simulink library "halin"  (R2021b)
settings: Solver=VariableStepAuto  StartTime=0.0  StopTime=10.0  RelTol=1e-3
undefined symbols (not defined in the file): TRUE
libraries: FVT_lib x177, hcu_lib x55
(part 15 of 17)

== system halin/HAL_IN/CAN3/MCU_B_R1/RrMCUDCBusCurr ==
  Rr_MCUDCBusCurr : Inport
  UnitConverter : DataTypeConversion  OutDataTypeStr=uint16
  convert_in : FVT_lib/hal/convert_in  gain=0.1  offset=-1500
  VHAL_RrMCUDCBusCurr_A : Outport
  wires:
  convert_in/1 -> VHAL_RrMCUDCBusCurr_A/1
  UnitConverter/1 -> convert_in/1
  Rr_MCUDCBusCurr/1 -> UnitConverter/1

== system halin/HAL_IN/CAN3/MCU_B_R1/RrMCUDCBusVolt ==
  Rr_MCUDCBusVolt : Inport
  UnitConverter : DataTypeConversion  OutDataTypeStr=uint16
  convert_in : FVT_lib/hal/convert_in  gain=0.1  offset=0
  VHAL_RrMCUDCBusVolt_V : Outport
  wires:
  convert_in/1 -> VHAL_RrMCUDCBusVolt_V/1
  UnitConverter/1 -> convert_in/1
  Rr_MCUDCBusVolt/1 -> UnitConverter/1

== system halin/HAL_IN/CAN3/MCU_B_R1/RrMCUDischrgSta ==
  Rr_MCUDischrgSta : Inport
  UnitConverter : DataTypeConversion  OutDataTypeStr=uint8
  VHAL_RrMCUDischrgSta_flg : Outport
  wires:
  UnitConverter/1 -> VHAL_RrMCUDischrgSta_flg/1
  Rr_MCUDischrgSta/1 -> UnitConverter/1

== system halin/HAL_IN/CAN3/MCU_B_R1/RrMCUEnaSta ==
  Rr_MCUEnaSta : Inport
  UnitConverter : DataTypeConversion  OutDataTypeStr=uint8
  VHAL_RrMCUEnaSta_flg : Outport
  wires:
  UnitConverter/1 -> VHAL_RrMCUEnaSta_flg/1
  Rr_MCUEnaSta/1 -> UnitConverter/1

== system halin/HAL_IN/CAN3/MCU_B_R1/RrMCUErr ==
  Rr_MCUErr : Inport
  UnitConverter : DataTypeConversion  OutDataTypeStr=uint8
  VHAL_RrMCUErr_enum : Outport
  wires:
  UnitConverter/1 -> VHAL_RrMCUErr_enum/1
  Rr_MCUErr/1 -> UnitConverter/1

== system halin/HAL_IN/CAN3/MCU_B_R1/RrMCUIGNsta ==
  Rr_MCUIGN_sta : Inport
  UnitConverter : DataTypeConversion  OutDataTypeStr=uint8
  VHAL_RrMCUIGNsta_flg : Outport
  wires:
  UnitConverter/1 -> VHAL_RrMCUIGNsta_flg/1
  Rr_MCUIGN_sta/1 -> UnitConverter/1

== system halin/HAL_IN/CAN3/MCU_B_R1/RrMCUReady ==
  Rr_MCUReady : Inport
  UnitConverter : DataTypeConversion  OutDataTypeStr=uint8
  VHAL_RrMCUReady_flg : Outport
  wires:
  UnitConverter/1 -> VHAL_RrMCUReady_flg/1
  Rr_MCUReady/1 -> UnitConverter/1

== system halin/HAL_IN/CAN3/MCU_B_R1/RrMCUReady4Pre ==
  Rr_MCUReady4Pre : Inport
  UnitConverter : DataTypeConversion  OutDataTypeStr=uint8
  VHAL_RrMCUReady4Pre_flg : Outport
  wires:
  UnitConverter/1 -> VHAL_RrMCUReady4Pre_flg/1
  Rr_MCUReady4Pre/1 -> UnitConverter/1

== system halin/HAL_IN/CAN3/MCU_B_R1/RrMCUSysSta ==
  Rr_MCUSysSta : Inport
  UnitConverter : DataTypeConversion  OutDataTypeStr=uint8
  VHAL_RrMCUSysSta_enum : Outport
  wires:
  UnitConverter/1 -> VHAL_RrMCUSysSta_enum/1
  Rr_MCUSysSta/1 -> UnitConverter/1

== system halin/HAL_IN/CAN3/MCU_B_R1/RrMCUTemp ==
  Rr_MCUTemp : Inport
  UnitConverter : DataTypeConversion  OutDataTypeStr=uint16
  convert_in : FVT_lib/hal/convert_in  gain=1  offset=-40
  VHAL_RrMCUTemp_C : Outport
  wires:
  convert_in/1 -> VHAL_RrMCUTemp_C/1
  UnitConverter/1 -> convert_in/1
  Rr_MCUTemp/1 -> UnitConverter/1

== system halin/HAL_IN/CAN3/MCU_B_R1/RrMotorAvailTq ==
  Rr_MotorAvailTq : Inport
  UnitConverter : DataTypeConversion  OutDataTypeStr=uint16
  VHAL_RrMotorAvailTq_Nm : Outport
  wires:
  UnitConverter/1 -> VHAL_RrMotorAvailTq_Nm/1
  Rr_MotorAvailTq/1 -> UnitConverter/1

== system halin/HAL_IN/CAN3/MCU_B_R1/RrRegenAvailTq ==
  Rr_RegenAvailTq : Inport
  UnitConverter : DataTypeConversion  OutDataTypeStr=uint16
  convert_in : FVT_lib/hal/convert_in  gain=1  offset=-1022
  VHAL_RrRegenAvailTq_Nm : Outport
  wires:
  convert_in/1 -> VHAL_RrRegenAvailTq_Nm/1
  UnitConverter/1 -> convert_in/1
  Rr_RegenAvailTq/1 -> UnitConverter/1

== system halin/HAL_IN/CAN3/MCU_B_R1/RrTMSpd ==
  Rr_TMSpd : Inport
  UnitConverter : DataTypeConversion  OutDataTypeStr=uint16
  convert_in : FVT_lib/hal/convert_in  gain=1  offset=-18000
  VHAL_RrTMSpd_rpm : Outport
  wires:
  convert_in/1 -> VHAL_RrTMSpd_rpm/1
  UnitConverter/1 -> convert_in/1
  Rr_TMSpd/1 -> UnitConverter/1

== system halin/HAL_IN/CAN3/MCU_B_R1/RrTMTemp ==
  Rr_TMTemp : Inport
  UnitConverter : DataTypeConversion  OutDataTypeStr=uint16
  convert_in : FVT_lib/hal/convert_in  gain=1  offset=-40
  VHAL_RrTMTemp_C : Outport
  wires:
  convert_in/1 -> VHAL_RrTMTemp_C/1
  UnitConverter/1 -> convert_in/1
  Rr_TMTemp/1 -> UnitConverter/1

== system halin/HAL_IN/CAN3/MCU_B_R1/RrTMid ==
  Rr_TMid : Inport
  UnitConverter : DataTypeConversion  OutDataTypeStr=uint16
  convert_in : FVT_lib/hal/convert_in  gain=0.1  offset=-1500
  VHAL_RrTMid_A : Outport
  wires:
  convert_in/1 -> VHAL_RrTMid_A/1
  UnitConverter/1 -> convert_in/1
  Rr_TMid/1 -> UnitConverter/1

== system halin/HAL_IN/CAN3/MCU_B_R1/RrTMiq ==
  Rr_TMiq : Inport
  UnitConverter : DataTypeConversion  OutDataTypeStr=uint16
  convert_in : FVT_lib/hal/convert_in  gain=0.1  offset=-1500
  VHAL_RrTMiq_A : Outport
  wires:
  convert_in/1 -> VHAL_RrTMiq_A/1
  UnitConverter/1 -> convert_in/1
  Rr_TMiq/1 -> UnitConverter/1

== system halin/HAL_IN/CAN3/MCU_B_R2/MCUBRLLCTempWarnSta ==
  MCU_B_R_LLCTempWarn_Sta : Inport
  UnitConverter : DataTypeConversion  OutDataTypeStr=uint8
  VHAL_MCUBRLLCTempWarnSta_enum : Outport
  wires:
  UnitConverter/1 -> VHAL_MCUBRLLCTempWarnSta_enum/1
  MCU_B_R_LLCTempWarn_Sta/1 -> UnitConverter/1

== system halin/HAL_IN/CAN3/MCU_B_R2/RrCoolanttempReq ==
  Rr_CoolanttempReq : Inport
  UnitConverter : DataTypeConversion  OutDataTypeStr=uint16
  convert_in : FVT_lib/hal/convert_in  gain=1  offset=-40
  VHAL_RrCoolanttempReq_cnt : Outport
  wires:
  convert_in/1 -> VHAL_RrCoolanttempReq_cnt/1
  UnitConverter/1 -> convert_in/1
  Rr_CoolanttempReq/1 -> UnitConverter/1

== system halin/HAL_IN/CAN3/MCU_B_R2/RrFailcode1 ==
  Rr_Failcode1 : Inport
  UnitConverter : DataTypeConversion  OutDataTypeStr=uint8
  VHAL_RrFailcode1_enum : Outport
  wires:
  UnitConverter/1 -> VHAL_RrFailcode1_enum/1
  Rr_Failcode1/1 -> UnitConverter/1

== system halin/HAL_IN/CAN3/MCU_B_R2/RrFailcode2 ==
  Rr_Failcode2 : Inport
  UnitConverter : DataTypeConversion  OutDataTypeStr=uint8
  VHAL_RrFailcode2_enum : Outport
  wires:
  UnitConverter/1 -> VHAL_RrFailcode2_enum/1
  Rr_Failcode2/1 -> UnitConverter/1

== system halin/HAL_IN/CAN3/MCU_B_R2/RrFailcodehistory1 ==
  Rr_Failcodehistory1 : Inport
  UnitConverter : DataTypeConversion  OutDataTypeStr=uint8
  VHAL_RrFailcodehistory1_enum : Outport
  wires:
  UnitConverter/1 -> VHAL_RrFailcodehistory1_enum/1
  Rr_Failcodehistory1/1 -> UnitConverter/1

== system halin/HAL_IN/CAN3/MCU_B_R2/RrFailcodehistory2 ==
  Rr_Failcodehistory2 : Inport
  UnitConverter : DataTypeConversion  OutDataTypeStr=uint8
  VHAL_RrFailcodehistory2_enum : Outport
  wires:
  UnitConverter/1 -> VHAL_RrFailcodehistory2_enum/1
  Rr_Failcodehistory2/1 -> UnitConverter/1

== system halin/HAL_IN/CAN3/MCU_B_R2/RrLLCTemp ==
  Rr_LLCTemp : Inport
  UnitConverter : DataTypeConversion  OutDataTypeStr=uint16
  convert_in : FVT_lib/hal/convert_in  gain=1  offset=-40
  VHAL_RrLLCTemp_C : Outport
  wires:
  convert_in/1 -> VHAL_RrLLCTemp_C/1
  UnitConverter/1 -> convert_in/1
  Rr_LLCTemp/1 -> UnitConverter/1

== system halin/HAL_IN/CAN3/MCU_B_R2/RrLLCflowReq ==
  Rr_LLCflowReq : Inport
  UnitConverter : DataTypeConversion  OutDataTypeStr=uint8
  convert_in : FVT_lib/hal/convert_in  gain=0.25  offset=0
  VHAL_RrLLCflowReq_Lpmin : Outport
  wires:
  convert_in/1 -> VHAL_RrLLCflowReq_Lpmin/1
  UnitConverter/1 -> convert_in/1
  Rr_LLCflowReq/1 -> UnitConverter/1

== system halin/HAL_IN/CAN3/MCU_B_R2/RrMCU3HWVer ==
  Rr_MCU3_HW_Ver : Inport
  UnitConverter : DataTypeConversion  OutDataTypeStr=uint16
  VHAL_RrMCU3HWVer_enum : Outport
  wires:
  UnitConverter/1 -> VHAL_RrMCU3HWVer_enum/1
  Rr_MCU3_HW_Ver/1 -> UnitConverter/1

== system halin/HAL_IN/CAN3/MCU_B_R2/RrMCU3SWVer ==
  Rr_MCU3_SW_Ver : Inport
  UnitConverter : DataTypeConversion  OutDataTypeStr=uint16
  VHAL_RrMCU3SWVer_enum : Outport
  wires:
  UnitConverter/1 -> VHAL_RrMCU3SWVer_enum/1
  Rr_MCU3_SW_Ver/1 -> UnitConverter/1

== system halin/HAL_IN/CAN3/MCU_B_R2/RrMCUTempWarn ==
  Rr_MCUTempWarn : Inport
  UnitConverter : DataTypeConversion  OutDataTypeStr=uint8
  VHAL_RrMCUTempWarn_enum : Outport
  wires:
  UnitConverter/1 -> VHAL_RrMCUTempWarn_enum/1
  Rr_MCUTempWarn/1 -> UnitConverter/1

== system halin/HAL_IN/CAN3/MCU_B_R2/RrTMTempWarn ==
  Rr_TMTempWarn : Inport
  UnitConverter : DataTypeConversion  OutDataTypeStr=uint8
  VHAL_RrTMTempWarn_enum : Outport
  wires:
  UnitConverter/1 -> VHAL_RrTMTempWarn_enum/1
  Rr_TMTempWarn/1 -> UnitConverter/1

== system halin/HAL_IN/CAN3/MCU_N_F1/FrActvDmpDisabStaNidec ==
  Fr_ActvDmpDisabSta_Nidec : Inport
  UnitConverter : DataTypeConversion  OutDataTypeStr=uint8
  VHAL_FrActvDmpDisabStaNidec_flg : Outport
  wires:
  UnitConverter/1 -> VHAL_FrActvDmpDisabStaNidec_flg/1
  Fr_ActvDmpDisabSta_Nidec/1 -> UnitConverter/1

== system halin/HAL_IN/CAN3/MCU_N_F1/FrEDUDrtStaNidec ==
  Fr_EDUDrtSta_Nidec : Inport
  UnitConverter : DataTypeConversion  OutDataTypeStr=uint8
  VHAL_FrEDUDrtStaNidec_flg : Outport
  wires:
  UnitConverter/1 -> VHAL_FrEDUDrtStaNidec_flg/1
  Fr_EDUDrtSta_Nidec/1 -> UnitConverter/1

== system halin/HAL_IN/CAN3/MCU_N_F1/FrEDUOpratingStaNidec ==
  Fr_EDUOpratingSta_Nidec : Inport
  UnitConverter : DataTypeConversion  OutDataTypeStr=uint8
  VHAL_FrEDUOpratingStaNidec_flg : Outport
  wires:
  UnitConverter/1 -> VHAL_FrEDUOpratingStaNidec_flg/1
  Fr_EDUOpratingSta_Nidec/1 -> UnitConverter/1

== system halin/HAL_IN/CAN3/MCU_N_F1/FrEDURealTMTqNidec ==
  Fr_EDURealTMTq_Nidec : Inport
  UnitConverter : DataTypeConversion  OutDataTypeStr=uint16
  convert_in : FVT_lib/hal/convert_in  gain=1  offset=-1022
  VHAL_FrEDURealTMTqNidec_Nm : Outport
  wires:
  convert_in/1 -> VHAL_FrEDURealTMTqNidec_Nm/1
  UnitConverter/1 -> convert_in/1
  Fr_EDURealTMTq_Nidec/1 -> UnitConverter/1

== system halin/HAL_IN/CAN3/MCU_N_F1/FrEDURotateDirctionNidec ==
  Fr_EDURotateDirction_Nidec : Inport
  UnitConverter : DataTypeConversion  OutDataTypeStr=uint8
  VHAL_FrEDURotateDirctionNidec_enum : Outport
  wires:
  UnitConverter/1 -> VHAL_FrEDURotateDirctionNidec_enum/1
  Fr_EDURotateDirction_Nidec/1 -> UnitConverter/1

== system halin/HAL_IN/CAN3/MCU_N_F1/FrEDUTqReqFbkNidec ==
  Fr_EDUTqReqFbk_Nidec : Inport
  UnitConverter : DataTypeConversion  OutDataTypeStr=uint16
  convert_in : FVT_lib/hal/convert_in  gain=1  offset=-1022
  VHAL_FrEDUTqReqFbkNidec_Nm : Outport
  wires:
  convert_in/1 -> VHAL_FrEDUTqReqFbkNidec_Nm/1
  UnitConverter/1 -> convert_in/1
  Fr_EDUTqReqFbk_Nidec/1 -> UnitConverter/1

== system halin/HAL_IN/CAN3/MCU_N_F1/FrMCU1ChksumNidec ==
  Fr_MCU1Chksum_Nidec : Inport
  UnitConverter : DataTypeConversion  OutDataTypeStr=uint8
  VHAL_FrMCU1ChksumNidec_enum : Outport
  wires:
  UnitConverter/1 -> VHAL_FrMCU1ChksumNidec_enum/1
  Fr_MCU1Chksum_Nidec/1 -> UnitConverter/1

== system halin/HAL_IN/CAN3/MCU_N_F1/FrMCU1RolCntNidec ==
  Fr_MCU1RolCnt_Nidec : Inport
  UnitConverter : DataTypeConversion  OutDataTypeStr=uint8
  VHAL_FrMCU1RolCntNidec_enum : Outport
  wires:
  UnitConverter/1 -> VHAL_FrMCU1RolCntNidec_enum/1
  Fr_MCU1RolCnt_Nidec/1 -> UnitConverter/1

== system halin/HAL_IN/CAN3/MCU_N_F1/FrMCUBATNidec ==
  Fr_MCUBAT_Nidec : Inport
  UnitConverter : DataTypeConversion  OutDataTypeStr=uint8
  convert_in : FVT_lib/hal/convert_in  gain=0.1  offset=0
  VHAL_FrMCUBATNidec_V : Outport
  wires:
  convert_in/1 -> VHAL_FrMCUBATNidec_V/1
  UnitConverter/1 -> convert_in/1
  Fr_MCUBAT_Nidec/1 -> UnitConverter/1

== system halin/HAL_IN/CAN3/MCU_N_F1/FrMCUDCBusCurrNidec ==
  Fr_MCUDCBusCurr_Nidec : Inport
  UnitConverter : DataTypeConversion  OutDataTypeStr=uint16
  convert_in : FVT_lib/hal/convert_in  gain=0.1  offset=-1500
  VHAL_FrMCUDCBusCurrNidec_A : Outport
  wires:
  convert_in/1 -> VHAL_FrMCUDCBusCurrNidec_A/1
  UnitConverter/1 -> convert_in/1
  Fr_MCUDCBusCurr_Nidec/1 -> UnitConverter/1

== system halin/HAL_IN/CAN3/MCU_N_F1/FrMCUDCBusVoltNidec ==
  Fr_MCUDCBusVolt_Nidec : Inport
  UnitConverter : DataTypeConversion  OutDataTypeStr=uint16
  convert_in : FVT_lib/hal/convert_in  gain=0.1  offset=0
  VHAL_FrMCUDCBusVoltNidec_V : Outport
  wires:
  convert_in/1 -> VHAL_FrMCUDCBusVoltNidec_V/1
  UnitConverter/1 -> convert_in/1
  Fr_MCUDCBusVolt_Nidec/1 -> UnitConverter/1

== system halin/HAL_IN/CAN3/MCU_N_F1/FrMCUDischrgStaNidec ==
  Fr_MCUDischrgSta_Nidec : Inport
  UnitConverter : DataTypeConversion  OutDataTypeStr=uint8
  VHAL_FrMCUDischrgStaNidec_flg : Outport
  wires:
  UnitConverter/1 -> VHAL_FrMCUDischrgStaNidec_flg/1
  Fr_MCUDischrgSta_Nidec/1 -> UnitConverter/1

== system halin/HAL_IN/CAN3/MCU_N_F1/FrMCUEnaStaNidec ==
  Fr_MCUEnaSta_Nidec : Inport
  UnitConverter : DataTypeConversion  OutDataTypeStr=uint8
  VHAL_FrMCUEnaStaNidec_flg : Outport
  wires:
  UnitConverter/1 -> VHAL_FrMCUEnaStaNidec_flg/1
  Fr_MCUEnaSta_Nidec/1 -> UnitConverter/1

== system halin/HAL_IN/CAN3/MCU_N_F1/FrMCUErrNidec ==
  Fr_MCUErr_Nidec : Inport
  UnitConverter : DataTypeConversion  OutDataTypeStr=uint8
  VHAL_FrMCUErrNidec_enum : Outport
  wires:
  UnitConverter/1 -> VHAL_FrMCUErrNidec_enum/1
  Fr_MCUErr_Nidec/1 -> UnitConverter/1

== system halin/HAL_IN/CAN3/MCU_N_F1/FrMCUIGNstaNidec ==
  Fr_MCUIGN_sta_Nidec : Inport
  UnitConverter : DataTypeConversion  OutDataTypeStr=uint8
  VHAL_FrMCUIGNstaNidec_flg : Outport
  wires:
  UnitConverter/1 -> VHAL_FrMCUIGNstaNidec_flg/1
  Fr_MCUIGN_sta_Nidec/1 -> UnitConverter/1

== system halin/HAL_IN/CAN3/MCU_N_F1/FrMCUReady4PreNidec ==
  Fr_MCUReady4Pre_Nidec : Inport
  UnitConverter : DataTypeConversion  OutDataTypeStr=uint8
  VHAL_FrMCUReady4PreNidec_flg : Outport
  wires:
  UnitConverter/1 -> VHAL_FrMCUReady4PreNidec_flg/1
  Fr_MCUReady4Pre_Nidec/1 -> UnitConverter/1

== system halin/HAL_IN/CAN3/MCU_N_F1/FrMCUReadyNidec ==
  Fr_MCUReady_Nidec : Inport
  UnitConverter : DataTypeConversion  OutDataTypeStr=uint8
  VHAL_FrMCUReadyNidec_flg : Outport
  wires:
  UnitConverter/1 -> VHAL_FrMCUReadyNidec_flg/1
  Fr_MCUReady_Nidec/1 -> UnitConverter/1

== system halin/HAL_IN/CAN3/MCU_N_F1/FrMCUSysStaNidec ==
  Fr_MCUSysSta_Nidec : Inport
  UnitConverter : DataTypeConversion  OutDataTypeStr=uint8
  VHAL_FrMCUSysStaNidec_enum : Outport
  wires:
  UnitConverter/1 -> VHAL_FrMCUSysStaNidec_enum/1
  Fr_MCUSysSta_Nidec/1 -> UnitConverter/1

== system halin/HAL_IN/CAN3/MCU_N_F1/FrMCUTempNidec ==
  Fr_MCUTemp_Nidec : Inport
  UnitConverter : DataTypeConversion  OutDataTypeStr=uint16
  convert_in : FVT_lib/hal/convert_in  gain=1  offset=-40
  VHAL_FrMCUTempNidec_C : Outport
  wires:
  convert_in/1 -> VHAL_FrMCUTempNidec_C/1
  UnitConverter/1 -> convert_in/1
  Fr_MCUTemp_Nidec/1 -> UnitConverter/1

== system halin/HAL_IN/CAN3/MCU_N_F1/FrMotorAvailTqNidec ==
  Fr_MotorAvailTq_Nidec : Inport
  UnitConverter : DataTypeConversion  OutDataTypeStr=uint16
  VHAL_FrMotorAvailTqNidec_Nm : Outport
  wires:
  UnitConverter/1 -> VHAL_FrMotorAvailTqNidec_Nm/1
  Fr_MotorAvailTq_Nidec/1 -> UnitConverter/1

== system halin/HAL_IN/CAN3/MCU_N_F1/FrRegenAvailTqNidec ==
  Fr_RegenAvailTq_Nidec : Inport
  UnitConverter : DataTypeConversion  OutDataTypeStr=uint16
  convert_in : FVT_lib/hal/convert_in  gain=1  offset=-1022
  VHAL_FrRegenAvailTqNidec_Nm : Outport
  wires:
  convert_in/1 -> VHAL_FrRegenAvailTqNidec_Nm/1
  UnitConverter/1 -> convert_in/1
  Fr_RegenAvailTq_Nidec/1 -> UnitConverter/1

== system halin/HAL_IN/CAN3/MCU_N_F1/FrTMSpdNidec ==
  Fr_TMSpd_Nidec : Inport
  UnitConverter : DataTypeConversion  OutDataTypeStr=uint16
  convert_in : FVT_lib/hal/convert_in  gain=1  offset=-17000
  VHAL_FrTMSpdNidec_rpm : Outport
  wires:
  convert_in/1 -> VHAL_FrTMSpdNidec_rpm/1
  UnitConverter/1 -> convert_in/1
  Fr_TMSpd_Nidec/1 -> UnitConverter/1

== system halin/HAL_IN/CAN3/MCU_N_F1/FrTMTempNidec ==
  Fr_TMTemp_Nidec : Inport
  UnitConverter : DataTypeConversion  OutDataTypeStr=uint16
  convert_in : FVT_lib/hal/convert_in  gain=1  offset=-40
  VHAL_FrTMTempNidec_C : Outport
  wires:
  convert_in/1 -> VHAL_FrTMTempNidec_C/1
  UnitConverter/1 -> convert_in/1
  Fr_TMTemp_Nidec/1 -> UnitConverter/1

== system halin/HAL_IN/CAN3/MCU_N_F1/FrTMidNidec ==
  Fr_TMid_Nidec : Inport
  UnitConverter : DataTypeConversion  OutDataTypeStr=uint16
  convert_in : FVT_lib/hal/convert_in  gain=0.1  offset=-1500
  VHAL_FrTMidNidec_A : Outport
  wires:
  convert_in/1 -> VHAL_FrTMidNidec_A/1
  UnitConverter/1 -> convert_in/1
  Fr_TMid_Nidec/1 -> UnitConverter/1

== system halin/HAL_IN/CAN3/MCU_N_F1/FrTMiqNidec ==
  Fr_TMiq_Nidec : Inport
  UnitConverter : DataTypeConversion  OutDataTypeStr=uint16
  convert_in : FVT_lib/hal/convert_in  gain=0.1  offset=-1500
  VHAL_FrTMiqNidec_A : Outport
  wires:
  convert_in/1 -> VHAL_FrTMiqNidec_A/1
  UnitConverter/1 -> convert_in/1
  Fr_TMiq_Nidec/1 -> UnitConverter/1

== system halin/HAL_IN/CAN3/MCU_N_F1/MCUWarnFNidec ==
  MCUWarn_F_Nidec : Inport
  UnitConverter : DataTypeConversion  OutDataTypeStr=uint8
  VHAL_MCUWarnFNidec_enum : Outport
  wires:
  UnitConverter/1 -> VHAL_MCUWarnFNidec_enum/1
  MCUWarn_F_Nidec/1 -> UnitConverter/1

== system halin/HAL_IN/CAN3/MCU_N_F2/FrCoolanttempReqNidec ==
  Fr_CoolanttempReq_Nidec : Inport
  UnitConverter : DataTypeConversion  OutDataTypeStr=uint16
  convert_in : FVT_lib/hal/convert_in  gain=1  offset=-40
  VHAL_FrCoolanttempReqNidec_C : Outport
  wires:
  convert_in/1 -> VHAL_FrCoolanttempReqNidec_C/1
  UnitConverter/1 -> convert_in/1
  Fr_CoolanttempReq_Nidec/1 -> UnitConverter/1

== system halin/HAL_IN/CAN3/MCU_N_F2/FrEOPSpdSetNidec ==
  Fr_EOP_SpdSet_Nidec : Inport
  UnitConverter : DataTypeConversion  OutDataTypeStr=uint16
  VHAL_FrEOPSpdSetNidec_rpm : Outport
  wires:
  UnitConverter/1 -> VHAL_FrEOPSpdSetNidec_rpm/1
  Fr_EOP_SpdSet_Nidec/1 -> UnitConverter/1

== system halin/HAL_IN/CAN3/MCU_N_F2/FrFailcode1Nidec ==
  Fr_Failcode1_Nidec : Inport
  UnitConverter : DataTypeConversion  OutDataTypeStr=uint8
  VHAL_FrFailcode1Nidec_enum : Outport
  wires:
  UnitConverter/1 -> VHAL_FrFailcode1Nidec_enum/1
  Fr_Failcode1_Nidec/1 -> UnitConverter/1

== system halin/HAL_IN/CAN3/MCU_N_F2/FrFailcode2Nidec ==
  Fr_Failcode2_Nidec : Inport
  UnitConverter : DataTypeConversion  OutDataTypeStr=uint8
  VHAL_FrFailcode2Nidec_enum : Outport
  wires:
  UnitConverter/1 -> VHAL_FrFailcode2Nidec_enum/1
  Fr_Failcode2_Nidec/1 -> UnitConverter/1

== system halin/HAL_IN/CAN3/MCU_N_F2/FrFailcodehistory1Nidec ==
  Fr_Failcodehistory1_Nidec : Inport
  UnitConverter : DataTypeConversion  OutDataTypeStr=uint8
  VHAL_FrFailcodehistory1Nidec_enum : Outport
  wires:
  UnitConverter/1 -> VHAL_FrFailcodehistory1Nidec_enum/1
  Fr_Failcodehistory1_Nidec/1 -> UnitConverter/1

== system halin/HAL_IN/CAN3/MCU_N_F2/FrFailcodehistory2Nidec ==
  Fr_Failcodehistory2_Nidec : Inport
  UnitConverter : DataTypeConversion  OutDataTypeStr=uint8
  VHAL_FrFailcodehistory2Nidec_enum : Outport
  wires:
  UnitConverter/1 -> VHAL_FrFailcodehistory2Nidec_enum/1
  Fr_Failcodehistory2_Nidec/1 -> UnitConverter/1

== system halin/HAL_IN/CAN3/MCU_N_F2/FrLLCTempNidec ==
  Fr_LLCTemp_Nidec : Inport
  UnitConverter : DataTypeConversion  OutDataTypeStr=uint16
  convert_in : FVT_lib/hal/convert_in  gain=1  offset=-40
  VHAL_FrLLCTempNidec_C : Outport
  wires:
  convert_in/1 -> VHAL_FrLLCTempNidec_C/1
  UnitConverter/1 -> convert_in/1
  Fr_LLCTemp_Nidec/1 -> UnitConverter/1

== system halin/HAL_IN/CAN3/MCU_N_F2/FrLLCflowReqNidec ==
  Fr_LLCflowReq_Nidec : Inport
  UnitConverter : DataTypeConversion  OutDataTypeStr=uint8
  convert_in : FVT_lib/hal/convert_in  gain=0.25  offset=0
  VHAL_FrLLCflowReqNidec_Lpmin : Outport
  wires:
  convert_in/1 -> VHAL_FrLLCflowReqNidec_Lpmin/1
  UnitConverter/1 -> convert_in/1
  Fr_LLCflowReq_Nidec/1 -> UnitConverter/1

== system halin/HAL_IN/CAN3/MCU_N_F2/FrMCUTempWarnNidec ==
  Fr_MCUTempWarn_Nidec : Inport
  UnitConverter : DataTypeConversion  OutDataTypeStr=uint8
  VHAL_FrMCUTempWarnNidec_enum : Outport
  wires:
  UnitConverter/1 -> VHAL_FrMCUTempWarnNidec_enum/1
  Fr_MCUTempWarn_Nidec/1 -> UnitConverter/1

== system halin/HAL_IN/CAN3/MCU_N_F2/FrTMTempWarnNidec ==
  Fr_TMTempWarn_Nidec : Inport
  UnitConverter : DataTypeConversion  OutDataTypeStr=uint8
  VHAL_FrTMTempWarnNidec_enum : Outport
  wires:
  UnitConverter/1 -> VHAL_FrTMTempWarnNidec_enum/1
  Fr_TMTempWarn_Nidec/1 -> UnitConverter/1

== system halin/HAL_IN/CAN3/MCU_N_F3/FrMCUHWVerNidec ==
  Fr_MCU_HW_Ver_Nidec : Inport
  UnitConverter : DataTypeConversion  OutDataTypeStr=uint16
  VHAL_FrMCUHWVerNidec_enum : Outport
  wires:
  UnitConverter/1 -> VHAL_FrMCUHWVerNidec_enum/1
  Fr_MCU_HW_Ver_Nidec/1 -> UnitConverter/1

== system halin/HAL_IN/CAN3/MCU_N_F3/FrMCUSWVerNidec ==
  Fr_MCU_SW_Ver_Nidec : Inport
  UnitConverter : DataTypeConversion  OutDataTypeStr=uint16
  VHAL_FrMCUSWVerNidec_enum : Outport
  wires:
  UnitConverter/1 -> VHAL_FrMCUSWVerNidec_enum/1
  Fr_MCU_SW_Ver_Nidec/1 -> UnitConverter/1

== system halin/HAL_IN/CAN3/MCU_N_R1/MCUWarnRNidec ==
  MCUWarn_R_Nidec : Inport
  UnitConverter : DataTypeConversion  OutDataTypeStr=uint8
  VHAL_MCUWarnRNidec_enum : Outport
  wires:
  UnitConverter/1 -> VHAL_MCUWarnRNidec_enum/1
  MCUWarn_R_Nidec/1 -> UnitConverter/1

== system halin/HAL_IN/CAN3/MCU_N_R1/RrActvDmpDisabStaNidec ==
  Rr_ActvDmpDisabSta_Nidec : Inport
  UnitConverter : DataTypeConversion  OutDataTypeStr=uint8
  VHAL_RrActvDmpDisabStaNidec_flg : Outport
  wires:
  UnitConverter/1 -> VHAL_RrActvDmpDisabStaNidec_flg/1
  Rr_ActvDmpDisabSta_Nidec/1 -> UnitConverter/1

== system halin/HAL_IN/CAN3/MCU_N_R1/RrEDUDrtStaNidec ==
  Rr_EDUDrtSta_Nidec : Inport
  UnitConverter : DataTypeConversion  OutDataTypeStr=uint8
  VHAL_RrEDUDrtStaNidec_flg : Outport
  wires:
  UnitConverter/1 -> VHAL_RrEDUDrtStaNidec_flg/1
  Rr_EDUDrtSta_Nidec/1 -> UnitConverter/1

== system halin/HAL_IN/CAN3/MCU_N_R1/RrEDUOpratingStaNidec ==
  Rr_EDUOpratingSta_Nidec : Inport
  UnitConverter : DataTypeConversion  OutDataTypeStr=uint8
  VHAL_RrEDUOpratingStaNidec_flg : Outport
  wires:
  UnitConverter/1 -> VHAL_RrEDUOpratingStaNidec_flg/1
  Rr_EDUOpratingSta_Nidec/1 -> UnitConverter/1

== system halin/HAL_IN/CAN3/MCU_N_R1/RrEDURealTMTqNidec ==
  Rr_EDURealTMTq_Nidec : Inport
  UnitConverter : DataTypeConversion  OutDataTypeStr=uint16
  convert_in : FVT_lib/hal/convert_in  gain=1  offset=-1022
  VHAL_RrEDURealTMTqNidec_Nm : Outport
  wires:
  convert_in/1 -> VHAL_RrEDURealTMTqNidec_Nm/1
  UnitConverter/1 -> convert_in/1
  Rr_EDURealTMTq_Nidec/1 -> UnitConverter/1

== system halin/HAL_IN/CAN3/MCU_N_R1/RrEDURotateDirctionNidec ==
  Rr_EDURotateDirction_Nidec : Inport
  UnitConverter : DataTypeConversion  OutDataTypeStr=uint8
  VHAL_RrEDURotateDirctionNidec_enum : Outport
  wires:
  UnitConverter/1 -> VHAL_RrEDURotateDirctionNidec_enum/1
  Rr_EDURotateDirction_Nidec/1 -> UnitConverter/1

== system halin/HAL_IN/CAN3/MCU_N_R1/RrEDUTqReqFbkNidec ==
  Rr_EDUTqReqFbk_Nidec : Inport
  UnitConverter : DataTypeConversion  OutDataTypeStr=uint16
  convert_in : FVT_lib/hal/convert_in  gain=1  offset=-1022
  VHAL_RrEDUTqReqFbkNidec_Nm : Outport
  wires:
  convert_in/1 -> VHAL_RrEDUTqReqFbkNidec_Nm/1
  UnitConverter/1 -> convert_in/1
  Rr_EDUTqReqFbk_Nidec/1 -> UnitConverter/1

== system halin/HAL_IN/CAN3/MCU_N_R1/RrMCU1ChksumNidec ==
  Rr_MCU1Chksum_Nidec : Inport
  UnitConverter : DataTypeConversion  OutDataTypeStr=uint8
  VHAL_RrMCU1ChksumNidec_enum : Outport
  wires:
  UnitConverter/1 -> VHAL_RrMCU1ChksumNidec_enum/1
  Rr_MCU1Chksum_Nidec/1 -> UnitConverter/1

== system halin/HAL_IN/CAN3/MCU_N_R1/RrMCU1RolCntNidec ==
  Rr_MCU1RolCnt_Nidec : Inport
  UnitConverter : DataTypeConversion  OutDataTypeStr=uint8
  VHAL_RrMCU1RolCntNidec_enum : Outport
  wires:
  UnitConverter/1 -> VHAL_RrMCU1RolCntNidec_enum/1
  Rr_MCU1RolCnt_Nidec/1 -> UnitConverter/1

== system halin/HAL_IN/CAN3/MCU_N_R1/RrMCUBATNidec ==
  Rr_MCUBAT_Nidec : Inport
  UnitConverter : DataTypeConversion  OutDataTypeStr=uint8
  convert_in : FVT_lib/hal/convert_in  gain=0.1  offset=0
  VHAL_RrMCUBATNidec_V : Outport
  wires:
  convert_in/1 -> VHAL_RrMCUBATNidec_V/1
  UnitConverter/1 -> convert_in/1
  Rr_MCUBAT_Nidec/1 -> UnitConverter/1

== system halin/HAL_IN/CAN3/MCU_N_R1/RrMCUDCBusCurrNidec ==
  Rr_MCUDCBusCurr_Nidec : Inport
  UnitConverter : DataTypeConversion  OutDataTypeStr=uint16
  convert_in : FVT_lib/hal/convert_in  gain=0.1  offset=-1500
  VHAL_RrMCUDCBusCurrNidec_A : Outport
  wires:
  convert_in/1 -> VHAL_RrMCUDCBusCurrNidec_A/1
  UnitConverter/1 -> convert_in/1
  Rr_MCUDCBusCurr_Nidec/1 -> UnitConverter/1

== system halin/HAL_IN/CAN3/MCU_N_R1/RrMCUDCBusVoltNidec ==
  Rr_MCUDCBusVolt_Nidec : Inport
  UnitConverter : DataTypeConversion  OutDataTypeStr=uint16
  convert_in : FVT_lib/hal/convert_in  gain=0.1  offset=0
  VHAL_RrMCUDCBusVoltNidec_V : Outport
  wires:
  convert_in/1 -> VHAL_RrMCUDCBusVoltNidec_V/1
  UnitConverter/1 -> convert_in/1
  Rr_MCUDCBusVolt_Nidec/1 -> UnitConverter/1

== system halin/HAL_IN/CAN3/MCU_N_R1/RrMCUDischrgStaNidec ==
  Rr_MCUDischrgSta_Nidec : Inport
  UnitConverter : DataTypeConversion  OutDataTypeStr=uint8
  VHAL_RrMCUDischrgStaNidec_flg : Outport
  wires:
  UnitConverter/1 -> VHAL_RrMCUDischrgStaNidec_flg/1
  Rr_MCUDischrgSta_Nidec/1 -> UnitConverter/1

== system halin/HAL_IN/CAN3/MCU_N_R1/RrMCUEnaStaNidec ==
  Rr_MCUEnaSta_Nidec : Inport
  UnitConverter : DataTypeConversion  OutDataTypeStr=uint8
  VHAL_RrMCUEnaStaNidec_flg : Outport
  wires:
  UnitConverter/1 -> VHAL_RrMCUEnaStaNidec_flg/1
  Rr_MCUEnaSta_Nidec/1 -> UnitConverter/1

== system halin/HAL_IN/CAN3/MCU_N_R1/RrMCUErrNidec ==
  Rr_MCUErr_Nidec : Inport
  UnitConverter : DataTypeConversion  OutDataTypeStr=uint8
  VHAL_RrMCUErrNidec_enum : Outport
  wires:
  UnitConverter/1 -> VHAL_RrMCUErrNidec_enum/1
  Rr_MCUErr_Nidec/1 -> UnitConverter/1

== system halin/HAL_IN/CAN3/MCU_N_R1/RrMCUIGNstaNidec ==
  Rr_MCUIGN_sta_Nidec : Inport
  UnitConverter : DataTypeConversion  OutDataTypeStr=uint8
  VHAL_RrMCUIGNstaNidec_flg : Outport
  wires:
  UnitConverter/1 -> VHAL_RrMCUIGNstaNidec_flg/1
  Rr_MCUIGN_sta_Nidec/1 -> UnitConverter/1

== system halin/HAL_IN/CAN3/MCU_N_R1/RrMCUReady4PreNidec ==
  Rr_MCUReady4Pre_Nidec : Inport
  UnitConverter : DataTypeConversion  OutDataTypeStr=uint8
  VHAL_RrMCUReady4PreNidec_flg : Outport
  wires:
  UnitConverter/1 -> VHAL_RrMCUReady4PreNidec_flg/1
  Rr_MCUReady4Pre_Nidec/1 -> UnitConverter/1

== system halin/HAL_IN/CAN3/MCU_N_R1/RrMCUReadyNidec ==
  Rr_MCUReady_Nidec : Inport
  UnitConverter : DataTypeConversion  OutDataTypeStr=uint8
  VHAL_RrMCUReadyNidec_flg : Outport
  wires:
  UnitConverter/1 -> VHAL_RrMCUReadyNidec_flg/1
  Rr_MCUReady_Nidec/1 -> UnitConverter/1

== system halin/HAL_IN/CAN3/MCU_N_R1/RrMCUSysStaNidec ==
  Rr_MCUSysSta_Nidec : Inport
  UnitConverter : DataTypeConversion  OutDataTypeStr=uint8
  VHAL_RrMCUSysStaNidec_enum : Outport
  wires:
  UnitConverter/1 -> VHAL_RrMCUSysStaNidec_enum/1
  Rr_MCUSysSta_Nidec/1 -> UnitConverter/1

== system halin/HAL_IN/CAN3/MCU_N_R1/RrMCUTempNidec ==
  Rr_MCUTemp_Nidec : Inport
  UnitConverter : DataTypeConversion  OutDataTypeStr=uint16
  convert_in : FVT_lib/hal/convert_in  gain=1  offset=-40
  VHAL_RrMCUTempNidec_C : Outport
  wires:
  convert_in/1 -> VHAL_RrMCUTempNidec_C/1
  UnitConverter/1 -> convert_in/1
  Rr_MCUTemp_Nidec/1 -> UnitConverter/1

== system halin/HAL_IN/CAN3/MCU_N_R1/RrMotorAvailTqNidec ==
  Rr_MotorAvailTq_Nidec : Inport
  UnitConverter : DataTypeConversion  OutDataTypeStr=uint16
  VHAL_RrMotorAvailTqNidec_Nm : Outport
  wires:
  UnitConverter/1 -> VHAL_RrMotorAvailTqNidec_Nm/1
  Rr_MotorAvailTq_Nidec/1 -> UnitConverter/1

== system halin/HAL_IN/CAN3/MCU_N_R1/RrRegenAvailTqNidec ==
  Rr_RegenAvailTq_Nidec : Inport
  UnitConverter : DataTypeConversion  OutDataTypeStr=uint16
  convert_in : FVT_lib/hal/convert_in  gain=1  offset=-1022
  VHAL_RrRegenAvailTqNidec_Nm : Outport
  wires:
  convert_in/1 -> VHAL_RrRegenAvailTqNidec_Nm/1
  UnitConverter/1 -> convert_in/1
  Rr_RegenAvailTq_Nidec/1 -> UnitConverter/1

== system halin/HAL_IN/CAN3/MCU_N_R1/RrTMSpdNidec ==
  Rr_TMSpd_Nidec : Inport
  UnitConverter : DataTypeConversion  OutDataTypeStr=uint16
  convert_in : FVT_lib/hal/convert_in  gain=1  offset=-17000
  VHAL_RrTMSpdNidec_rpm : Outport
  wires:
  convert_in/1 -> VHAL_RrTMSpdNidec_rpm/1
  UnitConverter/1 -> convert_in/1
  Rr_TMSpd_Nidec/1 -> UnitConverter/1

== system halin/HAL_IN/CAN3/MCU_N_R1/RrTMTempNidec ==
  Rr_TMTemp_Nidec : Inport
  UnitConverter : DataTypeConversion  OutDataTypeStr=uint16
  convert_in : FVT_lib/hal/convert_in  gain=1  offset=-40
  VHAL_RrTMTempNidec_C : Outport
  wires:
  convert_in/1 -> VHAL_RrTMTempNidec_C/1
  UnitConverter/1 -> convert_in/1
  Rr_TMTemp_Nidec/1 -> UnitConverter/1

== system halin/HAL_IN/CAN3/MCU_N_R1/RrTMidNidec ==
  Rr_TMid_Nidec : Inport
  UnitConverter : DataTypeConversion  OutDataTypeStr=uint16
  convert_in : FVT_lib/hal/convert_in  gain=0.1  offset=-1500
  VHAL_RrTMidNidec_A : Outport
  wires:
  convert_in/1 -> VHAL_RrTMidNidec_A/1
  UnitConverter/1 -> convert_in/1
  Rr_TMid_Nidec/1 -> UnitConverter/1

== system halin/HAL_IN/CAN3/MCU_N_R1/RrTMiqNidec ==
  Rr_TMiq_Nidec : Inport
  UnitConverter : DataTypeConversion  OutDataTypeStr=uint16
  convert_in : FVT_lib/hal/convert_in  gain=0.1  offset=-1500
  VHAL_RrTMiqNidec_A : Outport
  wires:
  convert_in/1 -> VHAL_RrTMiqNidec_A/1
  UnitConverter/1 -> convert_in/1
  Rr_TMiq_Nidec/1 -> UnitConverter/1

== system halin/HAL_IN/CAN3/MCU_N_R2/RrCoolanttempReqNidec ==
  Rr_CoolanttempReq_Nidec : Inport
  UnitConverter : DataTypeConversion  OutDataTypeStr=uint16
  convert_in : FVT_lib/hal/convert_in  gain=1  offset=-40
  VHAL_RrCoolanttempReqNidec_cnt : Outport
  wires:
  convert_in/1 -> VHAL_RrCoolanttempReqNidec_cnt/1
  UnitConverter/1 -> convert_in/1
  Rr_CoolanttempReq_Nidec/1 -> UnitConverter/1

== system halin/HAL_IN/CAN3/MCU_N_R2/RrEOPSpdSetNidec ==
  Rr_EOP_SpdSet_Nidec : Inport
  UnitConverter : DataTypeConversion  OutDataTypeStr=uint16
  VHAL_RrEOPSpdSetNidec_rpm : Outport
  wires:
  UnitConverter/1 -> VHAL_RrEOPSpdSetNidec_rpm/1
  Rr_EOP_SpdSet_Nidec/1 -> UnitConverter/1

== system halin/HAL_IN/CAN3/MCU_N_R2/RrFailcode1Nidec ==
  Rr_Failcode1_Nidec : Inport
  UnitConverter : DataTypeConversion  OutDataTypeStr=uint8
  VHAL_RrFailcode1Nidec_enum : Outport
  wires:
  UnitConverter/1 -> VHAL_RrFailcode1Nidec_enum/1
  Rr_Failcode1_Nidec/1 -> UnitConverter/1

== system halin/HAL_IN/CAN3/MCU_N_R2/RrFailcode2Nidec ==
  Rr_Failcode2_Nidec : Inport
  UnitConverter : DataTypeConversion  OutDataTypeStr=uint8
  VHAL_RrFailcode2Nidec_enum : Outport
  wires:
  UnitConverter/1 -> VHAL_RrFailcode2Nidec_enum/1
  Rr_Failcode2_Nidec/1 -> UnitConverter/1

== system halin/HAL_IN/CAN3/MCU_N_R2/RrFailcodehistory1Nidec ==
  Rr_Failcodehistory1_Nidec : Inport
  UnitConverter : DataTypeConversion  OutDataTypeStr=uint8
  VHAL_RrFailcodehistory1Nidec_enum : Outport
  wires:
  UnitConverter/1 -> VHAL_RrFailcodehistory1Nidec_enum/1
  Rr_Failcodehistory1_Nidec/1 -> UnitConverter/1

== system halin/HAL_IN/CAN3/MCU_N_R2/RrFailcodehistory2Nidec ==
  Rr_Failcodehistory2_Nidec : Inport
  UnitConverter : DataTypeConversion  OutDataTypeStr=uint8
  VHAL_RrFailcodehistory2Nidec_enum : Outport
  wires:
  UnitConverter/1 -> VHAL_RrFailcodehistory2Nidec_enum/1
  Rr_Failcodehistory2_Nidec/1 -> UnitConverter/1

== system halin/HAL_IN/CAN3/MCU_N_R2/RrLLCTempNidec ==
  Rr_LLCTemp_Nidec : Inport
  UnitConverter : DataTypeConversion  OutDataTypeStr=uint16
  convert_in : FVT_lib/hal/convert_in  gain=1  offset=-40
  VHAL_RrLLCTempNidec_C : Outport
  wires:
  convert_in/1 -> VHAL_RrLLCTempNidec_C/1
  UnitConverter/1 -> convert_in/1
  Rr_LLCTemp_Nidec/1 -> UnitConverter/1

== system halin/HAL_IN/CAN3/MCU_N_R2/RrLLCflowReqNidec ==
  Rr_LLCflowReq_Nidec : Inport
  UnitConverter : DataTypeConversion  OutDataTypeStr=uint8
  convert_in : FVT_lib/hal/convert_in  gain=0.25  offset=0
  VHAL_RrLLCflowReqNidec_Lpmin : Outport
  wires:
  convert_in/1 -> VHAL_RrLLCflowReqNidec_Lpmin/1
  UnitConverter/1 -> convert_in/1
  Rr_LLCflowReq_Nidec/1 -> UnitConverter/1

== system halin/HAL_IN/CAN3/MCU_N_R2/RrMCUTempWarnNidec ==
  Rr_MCUTempWarn_Nidec : Inport
  UnitConverter : DataTypeConversion  OutDataTypeStr=uint8
  VHAL_RrMCUTempWarnNidec_enum : Outport
  wires:
  UnitConverter/1 -> VHAL_RrMCUTempWarnNidec_enum/1
  Rr_MCUTempWarn_Nidec/1 -> UnitConverter/1

== system halin/HAL_IN/CAN3/MCU_N_R2/RrTMTempWarnNidec ==
  Rr_TMTempWarn_Nidec : Inport
  UnitConverter : DataTypeConversion  OutDataTypeStr=uint8
  VHAL_RrTMTempWarnNidec_enum : Outport
  wires:
  UnitConverter/1 -> VHAL_RrTMTempWarnNidec_enum/1
  Rr_TMTempWarn_Nidec/1 -> UnitConverter/1

== system halin/HAL_IN/CAN3/MCU_N_R3/RrMCU3HWVerNidec ==
  Rr_MCU3_HW_Ver_Nidec : Inport
  UnitConverter : DataTypeConversion  OutDataTypeStr=uint16
  VHAL_RrMCU3HWVerNidec_enum : Outport
  wires:
  UnitConverter/1 -> VHAL_RrMCU3HWVerNidec_enum/1
  Rr_MCU3_HW_Ver_Nidec/1 -> UnitConverter/1

== system halin/HAL_IN/CAN3/MCU_N_R3/RrMCU3SWVerNidec ==
  Rr_MCU3_SW_Ver_Nidec : Inport
  UnitConverter : DataTypeConversion  OutDataTypeStr=uint16
  VHAL_RrMCU3SWVerNidec_enum : Outport
  wires:
  UnitConverter/1 -> VHAL_RrMCU3SWVerNidec_enum/1
  Rr_MCU3_SW_Ver_Nidec/1 -> UnitConverter/1

== system halin/HAL_IN/CAN3/Shifter1/ShifterCRC8 ==
  Shifter_CRC8 : Inport
  UnitConverter : DataTypeConversion  OutDataTypeStr=uint8
  VHAL_ShifterCRC8_enum : Outport
  wires:
  UnitConverter/1 -> VHAL_ShifterCRC8_enum/1
  Shifter_CRC8/1 -> UnitConverter/1

== system halin/HAL_IN/CAN3/Shifter1/ShifterFailsta ==
  Shifter_Fail_sta : Inport
  UnitConverter : DataTypeConversion  OutDataTypeStr=uint8
  VHAL_ShifterFailsta_enum : Outport
  wires:
  UnitConverter/1 -> VHAL_ShifterFailsta_enum/1
  Shifter_Fail_sta/1 -> UnitConverter/1

== system halin/HAL_IN/CAN3/Shifter1/ShifterHandleCmd ==
  Shifter_Handle_Cmd : Inport
  UnitConverter : DataTypeConversion  OutDataTypeStr=uint8
  VHAL_ShifterHandleCmd_enum : Outport
  wires:
  UnitConverter/1 -> VHAL_ShifterHandleCmd_enum/1
  Shifter_Handle_Cmd/1 -> UnitConverter/1

== system halin/HAL_IN/CAN3/Shifter1/ShifterRC ==
  Shifter_RC : Inport
  UnitConverter : DataTypeConversion  OutDataTypeStr=uint8
  VHAL_ShifterRC_enum : Outport
  wires:
  UnitConverter/1 -> VHAL_ShifterRC_enum/1
  Shifter_RC/1 -> UnitConverter/1

== system halin/HAL_IN/CAN3/Shifter2/CSW2DimSwSta ==
  CSW2_DimSw_Sta : Inport
  UnitConverter : DataTypeConversion  OutDataTypeStr=uint8
  VHAL_CSW2DimSwSta_flg : Outport
  wires:
  UnitConverter/1 -> VHAL_CSW2DimSwSta_flg/1
  CSW2_DimSw_Sta/1 -> UnitConverter/1

== system halin/HAL_IN/CAN3/Shifter2/CSW2FWasSwSta ==
  CSW2_FWasSw_Sta : Inport
  UnitConverter : DataTypeConversion  OutDataTypeStr=uint8
  VHAL_CSW2FWasSwSta_enum : Outport
  wires:
  UnitConverter/1 -> VHAL_CSW2FWasSwSta_enum/1
  CSW2_FWasSw_Sta/1 -> UnitConverter/1

== system halin/HAL_IN/CAN3/Shifter2/CSW2FWipSwSta ==
  CSW2_FWipSw_Sta : Inport
  UnitConverter : DataTypeConversion  OutDataTypeStr=uint8
  VHAL_CSW2FWipSwSta_enum : Outport
  wires:
  UnitConverter/1 -> VHAL_CSW2FWipSwSta_enum/1
  CSW2_FWipSw_Sta/1 -> UnitConverter/1

== system halin/HAL_IN/CAN3/Shifter2/CSW2PassSWSta ==
  CSW2_PassSW_Sta : Inport
  UnitConverter : DataTypeConversion  OutDataTypeStr=uint8
  VHAL_CSW2PassSWSta_flg : Outport
  wires:
  UnitConverter/1 -> VHAL_CSW2PassSWSta_flg/1
  CSW2_PassSW_Sta/1 -> UnitConverter/1

== system halin/HAL_IN/CAN3/Shifter2/CSW2RWipWasSwSta ==
  CSW2_RWipWasSw_Sta : Inport
  UnitConverter : DataTypeConversion  OutDataTypeStr=uint8
  VHAL_CSW2RWipWasSwSta_enum : Outport
  wires:
  UnitConverter/1 -> VHAL_CSW2RWipWasSwSta_enum/1
  CSW2_RWipWasSw_Sta/1 -> UnitConverter/1

== system halin/HAL_IN/CAN3/Shifter2/CSW2TurnSwSta ==
  CSW2_TurnSw_Sta : Inport
  UnitConverter : DataTypeConversion  OutDataTypeStr=uint8
  VHAL_CSW2TurnSwSta_enum : Outport
  wires:
  UnitConverter/1 -> VHAL_CSW2TurnSwSta_enum/1
  CSW2_TurnSw_Sta/1 -> UnitConverter/1

== system halin/HAL_IN/CAN4/DKC1/DKCKeyNumSta ==
  DKC_KeyNum_Sta : Inport
  UnitConverter : DataTypeConversion  OutDataTypeStr=uint8
  VHAL_DKCKeyNumSta_enum : Outport
  wires:
  UnitConverter/1 -> VHAL_DKCKeyNumSta_enum/1
  DKC_KeyNum_Sta/1 -> UnitConverter/1

== system halin/HAL_IN/CAN4/DKC1/DKCKeyTypeSta ==
  DKC_KeyType_Sta : Inport
  UnitConverter : DataTypeConversion  OutDataTypeStr=uint8
  VHAL_DKCKeyTypeSta_enum : Outport
  wires:
  UnitConverter/1 -> VHAL_DKCKeyTypeSta_enum/1
  DKC_KeyType_Sta/1 -> UnitConverter/1

== system halin/HAL_IN/CAN4/DKC1/DKCPDkeyAreaRAPSSta ==
  DKC_PDkeyAreaRAPS_Sta : Inport
  UnitConverter : DataTypeConversion  OutDataTypeStr=uint8
  VHAL_DKCPDkeyAreaRAPSSta_enum : Outport
  wires:
  UnitConverter/1 -> VHAL_DKCPDkeyAreaRAPSSta_enum/1
  DKC_PDkeyAreaRAPS_Sta/1 -> UnitConverter/1

== system halin/HAL_IN/CAN4/DKC1/DKCParkingModeCmd ==
  DKC_ParkingMode_Cmd : Inport
  UnitConverter : DataTypeConversion  OutDataTypeStr=uint8
  VHAL_DKCParkingModeCmd_enum : Outport
  wires:
  UnitConverter/1 -> VHAL_DKCParkingModeCmd_enum/1
  DKC_ParkingMode_Cmd/1 -> UnitConverter/1

== system halin/HAL_IN/CAN4/DKC1/DKCReVehData ==
  DKC_Re_VehData : Inport
  UnitConverter : DataTypeConversion  OutDataTypeStr=uint8
  VHAL_DKCReVehData_enum : Outport
  wires:
  UnitConverter/1 -> VHAL_DKCReVehData_enum/1
  DKC_Re_VehData/1 -> UnitConverter/1

== system halin/HAL_IN/CAN4/DKC1/PCommandToBCM ==
  P_CommandToBCM : Inport
  UnitConverter : DataTypeConversion  OutDataTypeStr=uint8
  VHAL_PCommandToBCM_enum : Outport
  wires:
  UnitConverter/1 -> VHAL_PCommandToBCM_enum/1
  P_CommandToBCM/1 -> UnitConverter/1

== system halin/HAL_IN/CAN4/DKC1/PCommandToPTG ==
  P_CommandToPTG : Inport
  UnitConverter : DataTypeConversion  OutDataTypeStr=uint8
  VHAL_PCommandToPTG_enum : Outport
  wires:
  UnitConverter/1 -> VHAL_PCommandToPTG_enum/1
  P_CommandToPTG/1 -> UnitConverter/1

== system halin/HAL_IN/CAN4/DKC1/PDKeyAreaLockUnlock ==
  P_DKey_Area_LockUnlock : Inport
  UnitConverter : DataTypeConversion  OutDataTypeStr=uint8
  VHAL_PDKeyAreaLockUnlock_enum : Outport
  wires:
  UnitConverter/1 -> VHAL_PDKeyAreaLockUnlock_enum/1
  P_DKey_Area_LockUnlock/1 -> UnitConverter/1

== system halin/HAL_IN/CAN4/DKC1/PDKeyAreaPS ==
  P_DKey_Area_PS : Inport
  UnitConverter : DataTypeConversion  OutDataTypeStr=uint8
  VHAL_PDKeyAreaPS_enum : Outport
  wires:
  UnitConverter/1 -> VHAL_PDKeyAreaPS_enum/1
  P_DKey_Area_PS/1 -> UnitConverter/1

== system halin/HAL_IN/CAN4/DKC1/PDKeyAreaPTG ==
  P_DKey_Area_PTG : Inport
  UnitConverter : DataTypeConversion  OutDataTypeStr=uint8
  VHAL_PDKeyAreaPTG_enum : Outport
  wires:
  UnitConverter/1 -> VHAL_PDKeyAreaPTG_enum/1
  P_DKey_Area_PTG/1 -> UnitConverter/1

== system halin/HAL_IN/CAN4/DKC1/PDKeyWelcome ==
  P_DKey_Welcome : Inport
  UnitConverter : DataTypeConversion  OutDataTypeStr=uint8
  VHAL_PDKeyWelcome_enum : Outport
  wires:
  UnitConverter/1 -> VHAL_PDKeyWelcome_enum/1
  P_DKey_Welcome/1 -> UnitConverter/1

== system halin/HAL_IN/CAN4/DKC1/PDkeyShowIVI ==
  P_Dkey_Show_IVI : Inport
  UnitConverter : DataTypeConversion  OutDataTypeStr=uint8
  VHAL_PDkeyShowIVI_enum : Outport
  wires:
  UnitConverter/1 -> VHAL_PDkeyShowIVI_enum/1
  P_Dkey_Show_IVI/1 -> UnitConverter/1

== system halin/HAL_IN/CAN4/DKC1/PKeyMiss ==
  P_KeyMiss : Inport
  UnitConverter : DataTypeConversion  OutDataTypeStr=uint8
  VHAL_PKeyMiss_flg : Outport
  wires:
  UnitConverter/1 -> VHAL_PKeyMiss_flg/1
  P_KeyMiss/1 -> UnitConverter/1

== system halin/HAL_IN/CAN4/DKC1/PKeyMode ==
  P_KeyMode : Inport
  UnitConverter : DataTypeConversion  OutDataTypeStr=uint8
  VHAL_PKeyMode_enum : Outport
  wires:
  UnitConverter/1 -> VHAL_PKeyMode_enum/1
  P_KeyMode/1 -> UnitConverter/1

== system halin/HAL_IN/CAN4/DKC1/PUIDLowPower ==
  P_UID_LowPower : Inport
  UnitConverter : DataTypeConversion  OutDataTypeStr=uint8
  VHAL_PUIDLowPower_flg : Outport
  wires:
  UnitConverter/1 -> VHAL_PUIDLowPower_flg/1
  P_UID_LowPower/1 -> UnitConverter/1

== system halin/HAL_IN/CAN4/DKC2/EncryptionDATA063 ==
  EncryptionDATA_0_63 : Inport
  UnitConverter : DataTypeConversion  OutDataTypeStr=uint64
  VHAL_EncryptionDATA063_enum : Outport
  wires:
  UnitConverter/1 -> VHAL_EncryptionDATA063_enum/1
  EncryptionDATA_0_63/1 -> UnitConverter/1

== system halin/HAL_IN/CAN4/DKC2/EncryptionDATA64127 ==
  EncryptionDATA_64_127 : Inport
  UnitConverter : DataTypeConversion  OutDataTypeStr=uint64
  VHAL_EncryptionDATA64127_enum : Outport
  wires:
  UnitConverter/1 -> VHAL_EncryptionDATA64127_enum/1
  EncryptionDATA_64_127/1 -> UnitConverter/1

== system halin/HAL_IN/CAN4/DKC2/RandomNumberX ==
  Random_Number_X : Inport
  UnitConverter : DataTypeConversion  OutDataTypeStr=uint64
  VHAL_RandomNumberX_enum : Outport
  wires:
  UnitConverter/1 -> VHAL_RandomNumberX_enum/1
  Random_Number_X/1 -> UnitConverter/1

== system halin/HAL_IN/CAN4/PTG1/PTGActiveSta ==
  PTG_Active_Sta : Inport
  UnitConverter : DataTypeConversion  OutDataTypeStr=uint8
  VHAL_PTGActiveSta_enum : Outport
  wires:
  UnitConverter/1 -> VHAL_PTGActiveSta_enum/1
  PTG_Active_Sta/1 -> UnitConverter/1

== system halin/HAL_IN/CAN4/PTG1/PTGAutoStaus ==
  PTG_AutoStaus : Inport
  UnitConverter : DataTypeConversion  OutDataTypeStr=uint8
  VHAL_PTGAutoStaus_flg : Outport
  wires:
  UnitConverter/1 -> VHAL_PTGAutoStaus_flg/1
  PTG_AutoStaus/1 -> UnitConverter/1

== system halin/HAL_IN/CAN4/PTG1/PTGExist ==
  PTG_Exist : Inport
  UnitConverter : DataTypeConversion  OutDataTypeStr=uint8
  VHAL_PTGExist_flg : Outport
  wires:
  UnitConverter/1 -> VHAL_PTGExist_flg/1
  PTG_Exist/1 -> UnitConverter/1

== system halin/HAL_IN/CAN4/PTG1/PTGHWVer ==
  PTG_HW_Ver : Inport
  UnitConverter : DataTypeConversion  OutDataTypeStr=uint8
  VHAL_PTGHWVer_enum : Outport
  wires:
  UnitConverter/1 -> VHAL_PTGHWVer_enum/1
  PTG_HW_Ver/1 -> UnitConverter/1

== system halin/HAL_IN/CAN4/PTG1/PTGInnerSW2 ==
  PTG_Inner_SW_2 : Inport
  UnitConverter : DataTypeConversion  OutDataTypeStr=uint8
  VHAL_PTGInnerSW2_enum : Outport
  wires:
  UnitConverter/1 -> VHAL_PTGInnerSW2_enum/1
  PTG_Inner_SW_2/1 -> UnitConverter/1

== system halin/HAL_IN/CAN4/PTG1/PTGIsSetHeight ==
  PTG_Is_Set_Height : Inport
  UnitConverter : DataTypeConversion  OutDataTypeStr=uint8
  VHAL_PTGIsSetHeight_flg : Outport
  wires:
  UnitConverter/1 -> VHAL_PTGIsSetHeight_flg/1
  PTG_Is_Set_Height/1 -> UnitConverter/1

== system halin/HAL_IN/CAN4/PTG1/PTGRDILSta ==
  PTG_RDIL_Sta : Inport
  UnitConverter : DataTypeConversion  OutDataTypeStr=uint8
  VHAL_PTGRDILSta_enum : Outport
  wires:
  UnitConverter/1 -> VHAL_PTGRDILSta_enum/1
  PTG_RDIL_Sta/1 -> UnitConverter/1

== system halin/HAL_IN/CAN4/PTG1/PTGSWVer ==
  PTG_SW_Ver : Inport
  UnitConverter : DataTypeConversion  OutDataTypeStr=uint8
  VHAL_PTGSWVer_enum : Outport
  wires:
  UnitConverter/1 -> VHAL_PTGSWVer_enum/1
  PTG_SW_Ver/1 -> UnitConverter/1

== system halin/HAL_IN/CAN4/PTG1/PTGSysSta ==
  PTG_Sys_Sta : Inport
  UnitConverter : DataTypeConversion  OutDataTypeStr=uint8
  VHAL_PTGSysSta_enum : Outport
  wires:
  UnitConverter/1 -> VHAL_PTGSysSta_enum/1
  PTG_Sys_Sta/1 -> UnitConverter/1

== system halin/HAL_IN/CAN4/ZONE_DR1/DrLockSta ==
  DrLockSta : Inport
  UnitConverter : DataTypeConversion  OutDataTypeStr=uint8
  VHAL_DrLockSta_flg : Outport
  wires:
  UnitConverter/1 -> VHAL_DrLockSta_flg/1
  DrLockSta/1 -> UnitConverter/1

== system halin/HAL_IN/CAN4/ZONE_DR1/MIRRORFOLDSW ==
  MIRROR_FOLD_SW : Inport
  UnitConverter : DataTypeConversion  OutDataTypeStr=uint8
  VHAL_MIRRORFOLDSW_flg : Outport
  wires:
  UnitConverter/1 -> VHAL_MIRRORFOLDSW_flg/1
  MIRROR_FOLD_SW/1 -> UnitConverter/1

== system halin/HAL_IN/CAN4/ZONE_DR1/RLTurnLampC ==
  RLTurnLampC : Inport
  UnitConverter : DataTypeConversion  OutDataTypeStr=uint8
  convert_in : FVT_lib/hal/convert_in  gain=10  offset=0
  VHAL_RLTurnLampC_mA : Outport
  wires:
  convert_in/1 -> VHAL_RLTurnLampC_mA/1
  UnitConverter/1 -> convert_in/1
  RLTurnLampC/1 -> UnitConverter/1

== system halin/HAL_IN/CAN4/ZONE_DR1/RRTurnLampC ==
  RRTurnLampC : Inport
  UnitConverter : DataTypeConversion  OutDataTypeStr=uint8
  convert_in : FVT_lib/hal/convert_in  gain=10  offset=0
  VHAL_RRTurnLampC_mA : Outport
  wires:
  convert_in/1 -> VHAL_RRTurnLampC_mA/1
  UnitConverter/1 -> convert_in/1
  RRTurnLampC/1 -> UnitConverter/1

== system halin/HAL_IN/CAN4/ZONE_DR1/RWiperAS ==
  RWiperAS : Inport
  UnitConverter : DataTypeConversion  OutDataTypeStr=uint8
  VHAL_RWiperAS_flg : Outport
  wires:
  UnitConverter/1 -> VHAL_RWiperAS_flg/1
  RWiperAS/1 -> UnitConverter/1

== system halin/HAL_IN/CAN4/ZONE_DR1/RWiperProtection ==
  RWiperProtection : Inport
  UnitConverter : DataTypeConversion  OutDataTypeStr=uint8
  VHAL_RWiperProtection_flg : Outport
  wires:
  UnitConverter/1 -> VHAL_RWiperProtection_flg/1
  RWiperProtection/1 -> UnitConverter/1

== system halin/HAL_IN/CAN4/ZONE_DR_VCU/BlowerErr ==
  Blower_Err : Inport
  UnitConverter : DataTypeConversion  OutDataTypeStr=uint8
  VHAL_BlowerErr_enum : Outport
  wires:
  UnitConverter/1 -> VHAL_BlowerErr_enum/1
  Blower_Err/1 -> UnitConverter/1

== system halin/HAL_IN/CAN4/ZONE_DR_VCU/DrPMMLVOutPErrLmp ==
  DrPMMLVOutPErrLmp : Inport
  UnitConverter : DataTypeConversion  OutDataTypeStr=uint8
  VHAL_DrPMMLVOutPErrLmp_flg : Outport
  wires:
  UnitConverter/1 -> VHAL_DrPMMLVOutPErrLmp_flg/1
  DrPMMLVOutPErrLmp/1 -> UnitConverter/1

== system halin/HAL_IN/CAN4/ZONE_DR_VCU/DrPMMSysErrLmp ==
  DrPMMSysErrLmp : Inport
  UnitConverter : DataTypeConversion  OutDataTypeStr=uint8
  VHAL_DrPMMSysErrLmp_flg : Outport
  wires:
  UnitConverter/1 -> VHAL_DrPMMSysErrLmp_flg/1
  DrPMMSysErrLmp/1 -> UnitConverter/1

== system halin/HAL_IN/CAN4/ZONE_DR_VCU/DrSCPSysErrLmp ==
  DrSCPSysErrLmp : Inport
  UnitConverter : DataTypeConversion  OutDataTypeStr=uint8
  VHAL_DrSCPSysErrLmp_flg : Outport
  wires:
  UnitConverter/1 -> VHAL_DrSCPSysErrLmp_flg/1
  DrSCPSysErrLmp/1 -> UnitConverter/1

== system halin/HAL_IN/CAN4/ZONE_DR_VCU/DrStdAErrSta ==
  DrStdAErrSta : Inport
  UnitConverter : DataTypeConversion  OutDataTypeStr=uint8
  VHAL_DrStdAErrSta_flg : Outport
  wires:
  UnitConverter/1 -> VHAL_DrStdAErrSta_flg/1
  DrStdAErrSta/1 -> UnitConverter/1

== system halin/HAL_IN/CAN4/ZONE_DR_VCU/SolarL ==
  SolarL : Inport
  UnitConverter : DataTypeConversion  OutDataTypeStr=uint8
  convert_in : FVT_lib/hal/convert_in  gain=5  offset=0
  VHAL_SolarL_W : Outport
  wires:
  convert_in/1 -> VHAL_SolarL_W/1
  UnitConverter/1 -> convert_in/1
  SolarL/1 -> UnitConverter/1

== system halin/HAL_IN/CAN4/ZONE_DR_VCU/SolarLErr ==
  SolarL_Err : Inport
  UnitConverter : DataTypeConversion  OutDataTypeStr=uint8
  VHAL_SolarLErr_enum : Outport
  wires:
  UnitConverter/1 -> VHAL_SolarLErr_enum/1
  SolarL_Err/1 -> UnitConverter/1

== system halin/HAL_IN/CAN4/ZONE_DR_VCU/SolarR ==
  SolarR : Inport
  UnitConverter : DataTypeConversion  OutDataTypeStr=uint8
  convert_in : FVT_lib/hal/convert_in  gain=5  offset=0
  VHAL_SolarR_W : Outport
  wires:
  convert_in/1 -> VHAL_SolarR_W/1
  UnitConverter/1 -> convert_in/1
  SolarR/1 -> UnitConverter/1

== system halin/HAL_IN/CAN4/ZONE_DR_VCU/SolarRErr ==
  SolarR_Err : Inport
  UnitConverter : DataTypeConversion  OutDataTypeStr=uint8
  VHAL_SolarRErr_enum : Outport
  wires:
  UnitConverter/1 -> VHAL_SolarRErr_enum/1
  SolarR_Err/1 -> UnitConverter/1

== system halin/HAL_IN/CAN4/ZONE_DR_VCU/TFaceL ==
  T_Face_L : Inport
  UnitConverter : DataTypeConversion  OutDataTypeStr=uint8
  convert_in : FVT_lib/hal/convert_in  gain=0.5  offset=-40
  VHAL_TFaceL_C : Outport
  wires:
  convert_in/1 -> VHAL_TFaceL_C/1
  UnitConverter/1 -> convert_in/1
  T_Face_L/1 -> UnitConverter/1

== system halin/HAL_IN/CAN4/ZONE_DR_VCU/TFaceLErr ==
  T_Face_L_Err : Inport
  UnitConverter : DataTypeConversion  OutDataTypeStr=uint8
  VHAL_TFaceLErr_enum : Outport
  wires:
  UnitConverter/1 -> VHAL_TFaceLErr_enum/1
  T_Face_L_Err/1 -> UnitConverter/1

== system halin/HAL_IN/CAN4/ZONE_DR_VCU/TFaceR ==
  T_Face_R : Inport
  UnitConverter : DataTypeConversion  OutDataTypeStr=uint8
  convert_in : FVT_lib/hal/convert_in  gain=0.5  offset=-40
  VHAL_TFaceR_C : Outport
  wires:
  convert_in/1 -> VHAL_TFaceR_C/1
  UnitConverter/1 -> convert_in/1
  T_Face_R/1 -> UnitConverter/1

== system halin/HAL_IN/CAN4/ZONE_DR_VCU/TFaceRErr ==
  T_Face_R_Err : Inport
  UnitConverter : DataTypeConversion  OutDataTypeStr=uint8
  VHAL_TFaceRErr_enum : Outport
  wires:
  UnitConverter/1 -> VHAL_TFaceRErr_enum/1
  T_Face_R_Err/1 -> UnitConverter/1

== system halin/HAL_IN/CAN4/ZONE_DR_VCU/TFaceRr ==
  T_Face_Rr : Inport
  UnitConverter : DataTypeConversion  OutDataTypeStr=uint8
  convert_in : FVT_lib/hal/convert_in  gain=0.5  offset=-40
  VHAL_TFaceRr_C : Outport
  wires:
  convert_in/1 -> VHAL_TFaceRr_C/1
  UnitConverter/1 -> convert_in/1
  T_Face_Rr/1 -> UnitConverter/1

== system halin/HAL_IN/CAN4/ZONE_DR_VCU/TFaceRrErr ==
  T_Face_Rr_Err : Inport
  UnitConverter : DataTypeConversion  OutDataTypeStr=uint8
  VHAL_TFaceRrErr_enum : Outport
  wires:
  UnitConverter/1 -> VHAL_TFaceRrErr_enum/1
  T_Face_Rr_Err/1 -> UnitConverter/1

== system halin/HAL_IN/CAN4/ZONE_DR_VCU/TFootL ==
  T_Foot_L : Inport
  UnitConverter : DataTypeConversion  OutDataTypeStr=uint8
  convert_in : FVT_lib/hal/convert_in  gain=0.5  offset=-40
  VHAL_TFootL_C : Outport
  wires:
  convert_in/1 -> VHAL_TFootL_C/1
  UnitConverter/1 -> convert_in/1
  T_Foot_L/1 -> UnitConverter/1

== system halin/HAL_IN/CAN4/ZONE_DR_VCU/TFootLErr ==
  T_Foot_L_Err : Inport
  UnitConverter : DataTypeConversion  OutDataTypeStr=uint8
  VHAL_TFootLErr_enum : Outport
  wires:
  UnitConverter/1 -> VHAL_TFootLErr_enum/1
  T_Foot_L_Err/1 -> UnitConverter/1

== system halin/HAL_IN/CAN4/ZONE_DR_VCU/TFootR ==
  T_Foot_R : Inport
  UnitConverter : DataTypeConversion  OutDataTypeStr=uint8
  convert_in : FVT_lib/hal/convert_in  gain=0.5  offset=-40
  VHAL_TFootR_C : Outport
  wires:
  convert_in/1 -> VHAL_TFootR_C/1
  UnitConverter/1 -> convert_in/1
  T_Foot_R/1 -> UnitConverter/1
